simulink model "fuelcell"  (R2022b)
settings: Solver=VariableStepAuto  StartTime=0.0  StopTime=10720  RelTol=1e-2
model workspace (MAT data in the model file):
  N_P0 = 3
libraries: nesl_utility x7, sdl_lib x6, autolibshared x2, fl_lib x2, autolibrcnetworksystem x1, autolibmappedmotor x1
settings Model: Creator=connl  LastModifiedBy=user
settings SolverCC: MaxConsecutiveMinStep=5  DaesscMode=Robust  ZeroCrossAlgorithm=Adaptive  SolverResetMethod=Robust
settings DebuggingCC: AlgebraicLoopMsg=none  IgnoredZcDiagnostic=none

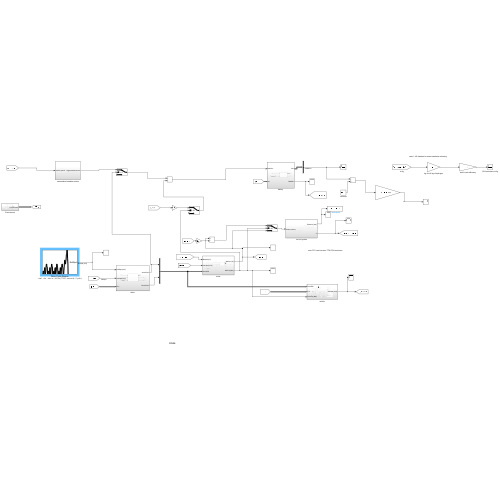
[thumbnail: Simulink's stored preview of the top-level diagram]
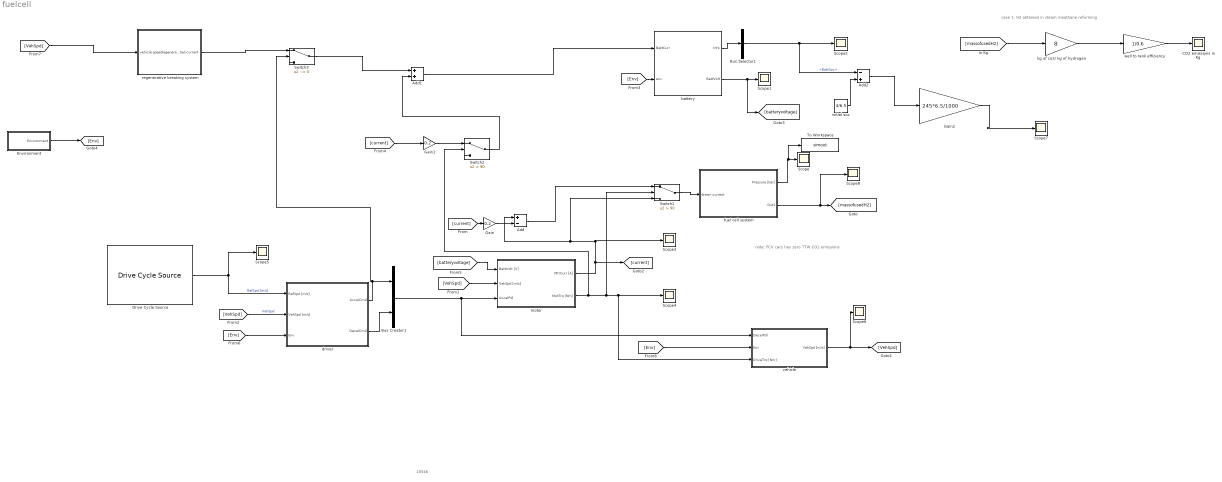
== system fuelcell ==
  note: 10546
  note: case 1: H2 obtained in steam meathane reforming
  note: note: FCV cars has zero TTW CO2 emissions
  Add : Sum  Inputs=+-
  Add1 : Sum
  Add2 : Sum  Inputs=-+
  Bus Creator1 : BusCreator  Inputs=2
  Bus Selector1 : BusSelector  OutputSignals=BattSoc
  CO2 emissions in Kg : Scope
  Drive Cycle Source : autolibshared/Drive Cycle Source  cycleVar=.mat, .xls, .xlsx or .txt file  wsVar=NEDC  fileVar=C:\Users\user\Desktop\my files\weekly meeting\drive cycles\NEDC.mat  tfinal="1180  seconds, Cyclic"  cycleRepeat=on  outAccPort=off  outGearPort=off  gearList=No gear data  t_wot1=5  xdot_woto=0  xdot_wot1=30  t_wot2=20  xdot_wot2=0  t_wotend=30  srcUnit=km/hr  outUnit=m/s  srcAccUnit=m/s/s  outAccUnit=m/s^2  dt=0  aMode=1  faultOption=off  velBnd=2  velBndUnit=mph  inUnit=m/s  timeBnd=1  failOption=off  stopSim=off  maxFaultCnt=10  maxFaultTime=2  maxTotFaultTime=15  traceOption=off  dtTrace=1  traceWindow=10  lastDCname=Custom Data Set 1  lastOutUnit=mph  lastDT=0  lastTB=1  lastSB=2  forceCalcBound=off
  Environment : Subsystem
  Gain : Gain  Gain=0.2
  Gain1 : Gain  Gain=0.2
  Gain2 : Gain  Gain=245*6.5/1000
  Scope{,1..8} (9 alike) : Scope
  Switch1 : Switch  Criteria=u2 > Threshold  Threshold=90  SaturateOnIntegerOverflow=off  InputSameDT=off
  Switch2 : Switch  Criteria=u2 > Threshold  Threshold=90  SaturateOnIntegerOverflow=off  InputSameDT=off
  Switch3 : Switch  Criteria=u2 ~= 0  SaturateOnIntegerOverflow=off  InputSameDT=off
  To Workspace : ToWorkspace  VariableName=simout  SaveFormat=Structure With Time  SampleTime=-1
  battery : Subsystem
  driver : Subsystem
  fuel cell system : Subsystem
  initial soc : Constant  Value=4/6.5
  kg of co2/ kg of hydrogen : Gain  Gain=8
  motor : Subsystem
  regenerative breaking system : Subsystem
  vehicle : Subsystem
  well to tank efficiency : Gain  Gain=1/0.6
  wires:
  Drive Cycle Source/1 -> Scope5/1, driver/1(RefSpd [m/s])  "RefSpd [m/s]"
  [VehSpd] -> driver/2(VehSpd [m/s])  "VehSpd"
  Bus Creator1/1 -> motor/3(AccelPdl), vehicle/1(DecelPdl)
  Environment/1(Environment) -> [Env]
  driver/2(DecelCmd) -> Bus Creator1/2
  driver/1(AccelCmd) -> Bus Creator1/1, Switch3/2
  [Env] -> driver/3(Env)
  fuel cell system/1(Pressure [bar]) -> To Workspace/1, Scope/1
  vehicle/1(VehSpd [m/s]) -> Scope6/1, [VehSpd]
  [Env] -> vehicle/2(Env)
  motor/2(MotTrq [Nm]) -> Switch1/2, Scope4/1, vehicle/3(DriveTrq [Nm]), Switch2/2
  [batteryvoltage] -> motor/1(BattVolt [V])
  [VehSpd] -> motor/2(VehSpd [m/s])
  [Env] -> battery/2(env)
  battery/1(Info) -> Bus Selector1/1
  motor/1(MtrCurr [A]) -> [current], Switch1/3, Add/1, Scope3/1
  Switch1/1 -> fuel cell system/1(drawn current)
  Add/1 -> Switch1/1
  Gain/1 -> Add/2
  Bus Selector1/1 -> Add2/1, Scope2/1  "<BattSoc>"
  [current] -> Gain/1
  [current] -> Gain1/1
  Gain1/1 -> Switch2/1
  Switch2/1 -> Add1/2
  [VehSpd] -> regenerative breaking system/1(vehicle speed)
  Switch3/1 -> Add1/1
  battery/2(BattVolt) -> [batteryvoltage], Scope1/1
  kg of co2/ kg of hydrogen/1 -> well to tank efficiency/1
  fuel cell system/2(Out1) -> Scope8/1, [massofusedH2]
  Add1/1 -> battery/1(BattCurr)
  well to tank efficiency/1 -> CO2 emissions in Kg/1
  [massofusedH2] -> kg of co2/ kg of hydrogen/1
  Add2/1 -> Gain2/1
  initial soc/1 -> Add2/2
  Gain2/1 -> Scope7/1
  regenerative breaking system/1(regenerated current) -> Switch3/1

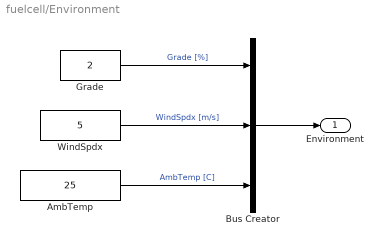
== system fuelcell/Environment ==
  AmbTemp : Constant  Value=25
  Bus Creator : BusCreator  Inputs=3
  Grade : Constant  Value=2
  WindSpdx : Constant  Value=5
  Environment : Outport
  wires:
  Grade/1 -> Bus Creator/1  "Grade [%]"
  WindSpdx/1 -> Bus Creator/2  "WindSpdx [m/s]"
  AmbTemp/1 -> Bus Creator/3  "AmbTemp [C]"
  Bus Creator/1 -> Environment/1

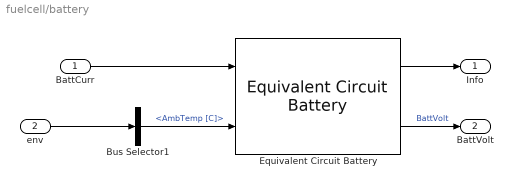
== system fuelcell/battery ==
  BattCurr : Inport
  env : Inport  Port=2
  Bus Selector1 : BusSelector  OutputSignals=AmbTemp [C]
  Equivalent Circuit Battery : autolibrcnetworksystem/Equivalent Circuit Battery  CapacityCtrl=Parameter  OutputVlt=Filtered  NumRC=1  Em=[245 245; 245 245]  R0=[0.011 0.11; 0.011 0.011]  SOC_BP=[0.5 1]  Temperature_BP=[293.15 313.15]  BattCap=[6.5 6.5]  BattCapInit=4  InitialCapVoltage=0  Tc=1/1000  Vinit=4.193  R1=[0.011 0.011; 0.011 0.011]  C1=|  R2=[0.011 0.011; 0.011 0.011]  C2=|  R3=[0.011 0.011; 0.011 0.011]  C3=|  R4=|  C4=|  R5=|  C5=|  Vu=Inf  Vl=-Inf  RefBlkName='autolibrcnetworksystem/Equivalent Circuit Battery'
      C1=|
      | [2287.7 11897;
      | 6122 24515]
      C2=|
      | [2287.7 11897;
      | 6122 24515]
      C3=|
      | [2287.7 11897;
      | 6122 24515]
      R4=|
      | [0.010342 0.0012244;
      | 0.0067316 0.0011396;
      | 0.0051156 0.0012661;
      | 0.0043447 0.0012265;
      | 0.0038826 0.0011163;
      | 0.0034226 0.0009968;
      | 0.003346 0.0011458;
      | 0.0033222 0.001345;
      | 0.0033201 0.0013091;
      | 0.0032886 0.0010986;
      | 0.0028114 0.0010309]
      C4=|
      | [2287.7 11897;
      | 6122 24515;
      | 18460 42098;
      | 20975 44453;
      | 15254 33098;
      | 10440 24492;
      | 13903 32975;
      | 16694 40007;
      | 15784 35937;
      | 12165 26430;
      | 9118 24795]
      R5=|
      | [0.010342 0.0012244;
      | 0.0067316 0.0011396;
      | 0.0051156 0.0012661;
      | 0.0043447 0.0012265;
      | 0.0038826 0.0011163;
      | 0.0034226 0.0009968;
      | 0.003346 0.0011458;
      | 0.0033222 0.001345;
      | 0.0033201 0.0013091;
      | 0.0032886 0.0010986;
      | 0.0028114 0.0010309]
      C5=|
      | [2287.7 11897;
      | 6122 24515;
      | 18460 42098;
      | 20975 44453;
      | 15254 33098;
      | 10440 24492;
      | 13903 32975;
      | 16694 40007;
      | 15784 35937;
      | 12165 26430;
      | 9118 24795]
  Info : Outport
  BattVolt : Outport  Port=2
  wires:
  Equivalent Circuit Battery/2 -> BattVolt/1  "BattVolt"
  env/1 -> Bus Selector1/1
  BattCurr/1 -> Equivalent Circuit Battery/1
  Equivalent Circuit Battery/1 -> Info/1
  Bus Selector1/1 -> Equivalent Circuit Battery/2  "<AmbTemp [C]>"

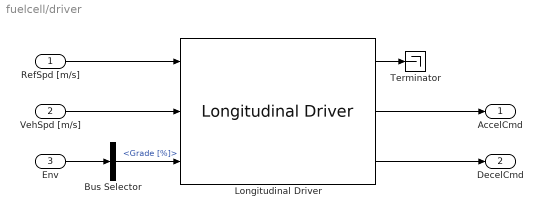
== system fuelcell/driver ==
  RefSpd [m/s] : Inport
  VehSpd [m/s] : Inport  Port=2
  Env : Inport  Port=3
  Bus Selector : BusSelector  OutputSignals=Grade [%]
  Longitudinal Driver : autolibshared/Longitudinal Driver  extAccelOvr=off  extDecelOvr=off  extAccelHld=off  extDecelHld=off  extAccelZero=off  extDecelZero=off  cntrlType=PI  shftType=None  velUnits=m/s  gearOut=off  Kp=10  Ki=2  Kff=0.05  Kg=0.01  VehVelVec=[0 100]  KffVec=[.1 .1]  KpVec=[10 10]  KiVec=[5 5]  KgVec=[0 0]  m=1500  Kpt=3000  tau=.1  L=2  aR=200  bR=2.5  cR=.5  g=9.81  vnom=100  Kaw=0.1  tauerr=0.03  tauPt=2  GearInit=0  tShift=.1  pdlVec=[0.1 0.4 0.5 0.9]  upShftTbl=[-1 12.9375 26.4375 39.9375 51.18749999999999 62.4375 72.84375 83.25;-1 16.3125 29.8125 43.3125 54.5624 65.8125 76.78125 87.75;-1 19.6875 33.1875 46.68749999999999 57.9375 69.1875 80.71875 92.25;-1 33 52.5 77.25 100.5 138.75 161.875 185]  dwnShftTbl=[1 9.5625 23.0625 36.5625 47.8125 59.0625 68.90625 78.75;1 12.9375 26.4375 39.9375 51.18749999999999 62.4375 72.84375 83.25;1 16.3125 29.8125 43.3125 54.562499 65.8125 76.78125 87.75;1 19.6875 33.1875 46.68749999999999 57.9375 69.1875 80.71875 92.25]  tClutch=.5  tRev=.5  tPark=120  aMode=1  UpGearVec="[0  1  2  3  4  5  6  7]"  DownGearVec="[1  2  3  4  5  6  7  8]"
  Terminator : Terminator
  AccelCmd : Outport
  DecelCmd : Outport  Port=2
  wires:
  Longitudinal Driver/1 -> Terminator/1
  Env/1 -> Bus Selector/1
  Bus Selector/1 -> Longitudinal Driver/3  "<Grade [%]>"
  RefSpd [m/s]/1 -> Longitudinal Driver/1
  VehSpd [m/s]/1 -> Longitudinal Driver/2
  Longitudinal Driver/3 -> DecelCmd/1
  Longitudinal Driver/2 -> AccelCmd/1

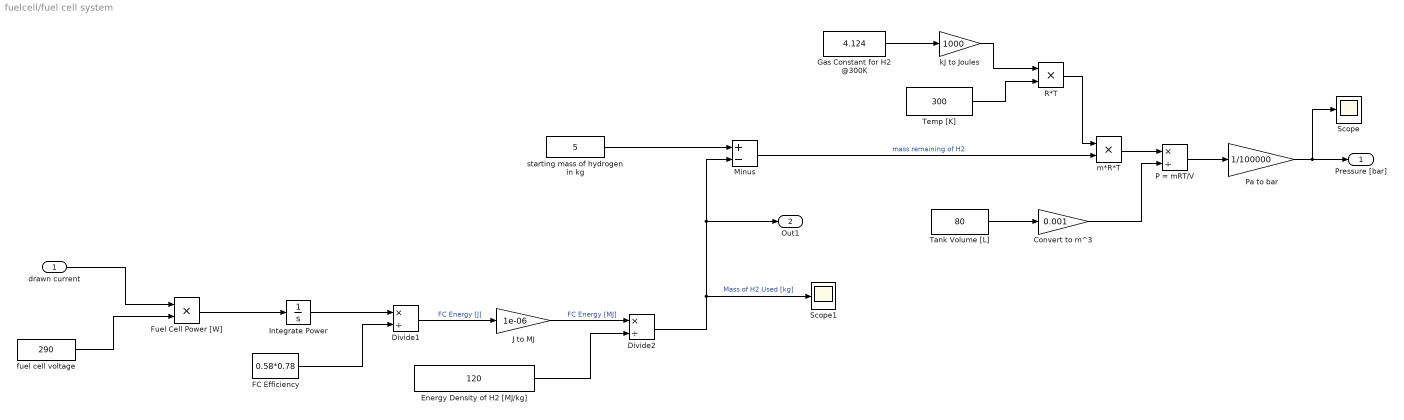
== system fuelcell/fuel cell system ==
  drawn current : Inport
  Convert to m^3 : Gain  Gain=0.001
  Divide1 : Product  Inputs=*/
  Divide2 : Product  Inputs=*/
  Energy Density of H2 [MJ/kg] : Constant  Value=120
  FC Efficiency : Constant  Value=0.58*0.78
  Fuel Cell Power [W] : Product
  Gas Constant for H2 @300K : Constant  Value=4.124
  Integrate Power : Integrator
  J to MJ : Gain  Gain=1e-06
  Minus : Sum  Inputs=+-
  P = mRT/V : Product  Inputs=*/
  Pa to bar : Gain  Gain=1/100000
  R*T : Product
  Scope : Scope
  Scope1 : Scope
  Tank Volume [L] : Constant  Value=80
  Temp [K] : Constant  Value=300
  fuel cell voltage : Constant  Value=290
  kJ to Joules : Gain  Gain=1000
  m*R*T : Product
  starting mass of hydrogen in kg : Constant  Value=5
  Pressure [bar] : Outport
  Out1 : Outport  Port=2
  wires:
  FC Efficiency/1 -> Divide1/2
  Integrate Power/1 -> Divide1/1
  m*R*T/1 -> P = mRT/V/1
  Pa to bar/1 -> Pressure [bar]/1, Scope/1
  P = mRT/V/1 -> Pa to bar/1
  fuel cell voltage/1 -> Fuel Cell Power [W]/2
  J to MJ/1 -> Divide2/1  "FC Energy [MJ]"
  drawn current/1 -> Fuel Cell Power [W]/1
  Gas Constant for H2 @300K/1 -> kJ to Joules/1
  Divide1/1 -> J to MJ/1  "FC Energy [J]"
  Minus/1 -> m*R*T/2  "mass remaining of H2"
  Divide2/1 -> Out1/1, Minus/2, Scope1/1  "Mass of H2 Used [kg]"
  kJ to Joules/1 -> R*T/1
  Convert to m^3/1 -> P = mRT/V/2
  R*T/1 -> m*R*T/1
  Tank Volume [L]/1 -> Convert to m^3/1
  Temp [K]/1 -> R*T/2
  Fuel Cell Power [W]/1 -> Integrate Power/1
  starting mass of hydrogen in kg/1 -> Minus/1
  Energy Density of H2 [MJ/kg]/1 -> Divide2/2

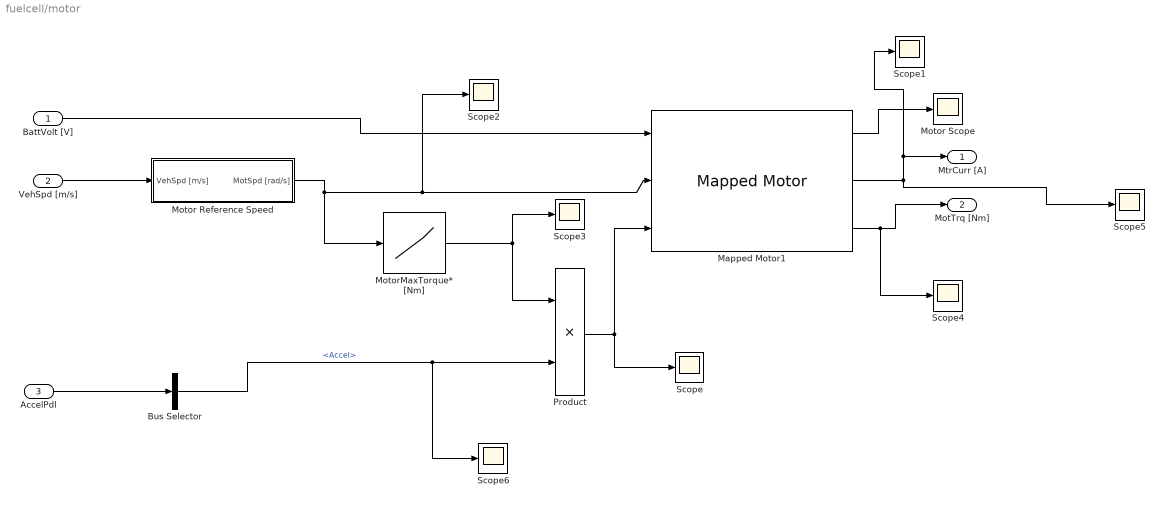
== system fuelcell/motor ==
  BattVolt [V] : Inport
  VehSpd [m/s] : Inport  Port=2
  AccelPdl : Inport  Port=3
  Bus Selector : BusSelector  OutputSignals=Accel
  Mapped Motor1 : autolibmappedmotor/Mapped Motor  port_config=Speed  param_by=Tabulated torque-speed envelope  w_t=[ 500 1000 1750 2000 3450]  T_t=[ 2494 1247 712 623 361]  torque_max=110  power_max=21000  Tc=0.02  param_loss=Single efficiency measurement  eff=90  w_eff=400  T_eff=55  Piron=0  Pbase=0  w_eff_bp=[-800 -400 0 400 800]  T_eff_bp=[0 0.03 0.06 0.09]  Temp_eff_bp=[233.15 293.15 373.15]  losses_table=[1.49 1.67 2.21 3.10; 0.42 0.69 1.14 2.03; 0.06 0.24 0.78 1.68; 0.42 0.69 1.14 2.03; 1.49 1.67 2.21 3.10]  losses_table_3d=cat(3,[1.49 1.67 2.21 3.10; 0.42 0.69 1.14 2.03; 0.06 0.24 0.78 1.68; 0.42 0.69 1.14 2.03; 1.49 1.67 2.21 3.10],[1.49 1.67 2.21 3.10; 0.42 0.69 1.14 2.03; 0.06 0.24 0.78 1.68; 0.42 0.69 1.14 2.03; 1.49 1.67 2.21 3.10],[1.49 1.67 2.21 3.10; 0.42 0.69 1.14 2.03; 0.06 0.24 0.78 1.68; 0.42 0.69 1.14 2.03; 1.49 1.67 2.21 3.10])  efficiency_table=[95 95 95 95; 95 95 95 95; 95 95 95 95; 95 95 95 95; 95 95 95 95]  efficiency_table_3d=cat(3,[95 95 95 95; 95 95 95 95; 95 95 95 95; 95 95 95 95; 95 95 95 95],[95 95 95 95; 95 95 95 95; 95 95 95 95; 95 95 95 95; 95 95 95 95],[95 95 95 95; 95 95 95 95; 95 95 95 95; 95 95 95 95; 95 95 95 95])  J=5e-6  b=1e-5  omega_o=0  T_t_extended=[361 623 712 1247 2494 2494 1247 712 623 361]  w_t_extended=[-3450 -2000 -1750 -1000 -500 500 1000 1750 2000 3450]  KLossIron=0  KLossCopper=0.80808  x_w_eff_vec=[-8000 -4000 0 4000 8000]  x_T_eff_vec=[-0.09 -0.06 -0.03 0 0.03 0.06 0.09]  x_tmp_eff_vec=[-0.09 -0.06 -0.03 0 0.03 0.06 0.09]  x_losses_mat=[3.1 2.21 1.67 1.49 1.67 2.21 3.1;2.03 1.14 0.69 0.42 0.69 1.14 2.03;1.68 0.78 0.24 0.06 0.24 0.78 1.68;2.03 1.14 0.69 0.42 0.69 1.14 2.03;3.1 2.21 1.67 1.49 1.67 2.21 3.1]  x_losses_mat_3d=[37.8947368421052 25.2631578947368 12.6315789473684 0 12 24 36;18.9473684210526 12.6315789473684 6.3157894736842 0 5.99999999999999 12 18;0 0 0 0 0 0 0;18 12 5.99999999999999 0 6.3157894736842 12.6315789473684 18.9473684210526;36 24 12 0 12.6315789473684 25.2631578947368 37.8947368421052]  CalLossMapData={}  CalLossWithTempMapData={}  aMode=1  RefBlkName='autolibmappedmotor/Mapped Motor'
  Motor Reference Speed : Subsystem
  Motor Scope : Scope
  MotorMaxTorque* [Nm] : Lookup_n-D  NumberOfTableDimensions=1  BreakpointsForDimension1=[ 500 1000 1750 2000 3450]  Table="[  2494 1247 712 623 361]"  InternalRulePriority=Speed  RndMeth=Simplest
  Product : Product
  Scope{,1..6} (7 alike) : Scope
  MtrCurr [A] : Outport
  MotTrq [Nm] : Outport  Port=2
  wires:
  Mapped Motor1/2 -> Scope1/1, MtrCurr [A]/1, Scope5/1
  Mapped Motor1/1 -> Motor Scope/1
  BattVolt [V]/1 -> Mapped Motor1/1
  Mapped Motor1/3 -> Scope4/1, MotTrq [Nm]/1
  Motor Reference Speed/1(MotSpd [rad/s]) -> Scope2/1, Mapped Motor1/2, MotorMaxTorque* [Nm]/1
  MotorMaxTorque* [Nm]/1 -> Product/1, Scope3/1
  VehSpd [m/s]/1 -> Motor Reference Speed/1(VehSpd [m/s])
  Bus Selector/1 -> Scope6/1, Product/2  "<Accel>"
  AccelPdl/1 -> Bus Selector/1
  Product/1 -> Mapped Motor1/3, Scope/1

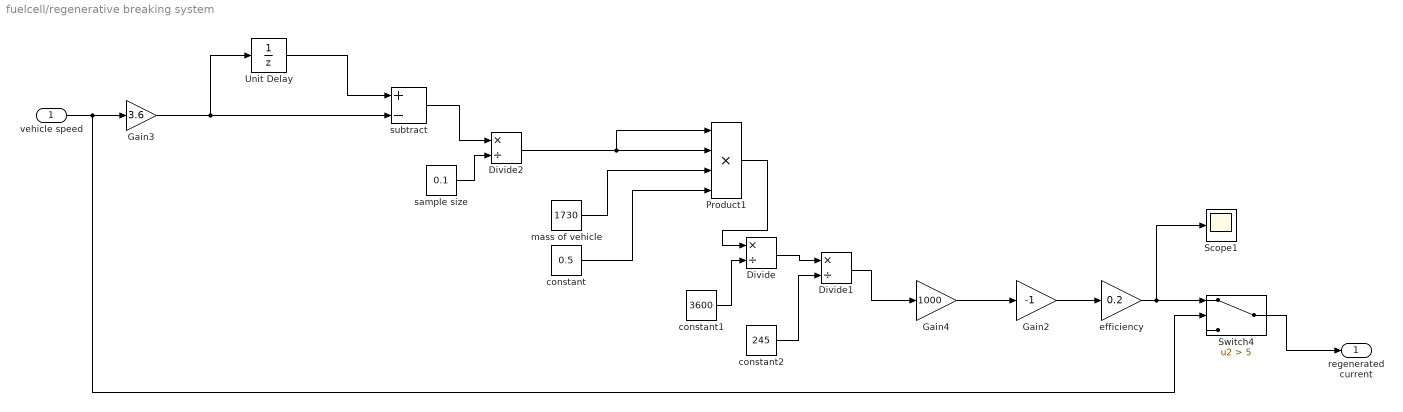
== system fuelcell/regenerative breaking system ==
  vehicle speed : Inport
  Divide : Product  Inputs=*/
  Divide1 : Product  Inputs=*/
  Divide2 : Product  Inputs=*/
  Gain2 : Gain  Gain=-1
  Gain3 : Gain  Gain=3.6
  Gain4 : Gain  Gain=1000
  Product1 : Product  Inputs=4
  Scope1 : Scope
  Switch4 : Switch  Criteria=u2 > Threshold  Threshold=5  SaturateOnIntegerOverflow=off  InputSameDT=off
  Unit Delay : UnitDelay  SampleTime=0.1  HasFrameUpgradeWarning=on
  constant : Constant  Value=0.5
  constant1 : Constant  Value=3600
  constant2 : Constant  Value=245
  efficiency : Gain  Gain=0.2
  mass of vehicle : Constant  Value=1730
  sample size : Constant  Value=0.1
  subtract : Sum  Inputs=+-
  regenerated current : Outport
  wires:
  constant1/1 -> Divide/2
  Divide1/1 -> Gain4/1
  constant2/1 -> Divide1/2
  mass of vehicle/1 -> Product1/3
  Gain3/1 -> subtract/2, Unit Delay/1
  Divide/1 -> Divide1/1
  Unit Delay/1 -> subtract/1
  constant/1 -> Product1/4
  Gain4/1 -> Gain2/1
  Switch4/1 -> regenerated current/1
  Gain2/1 -> efficiency/1
  efficiency/1 -> Scope1/1, Switch4/1
  Product1/1 -> Divide/1
  vehicle speed/1 -> Switch4/2, Gain3/1
  subtract/1 -> Divide2/1
  Divide2/1 -> Product1/2, Product1/1
  sample size/1 -> Divide2/2

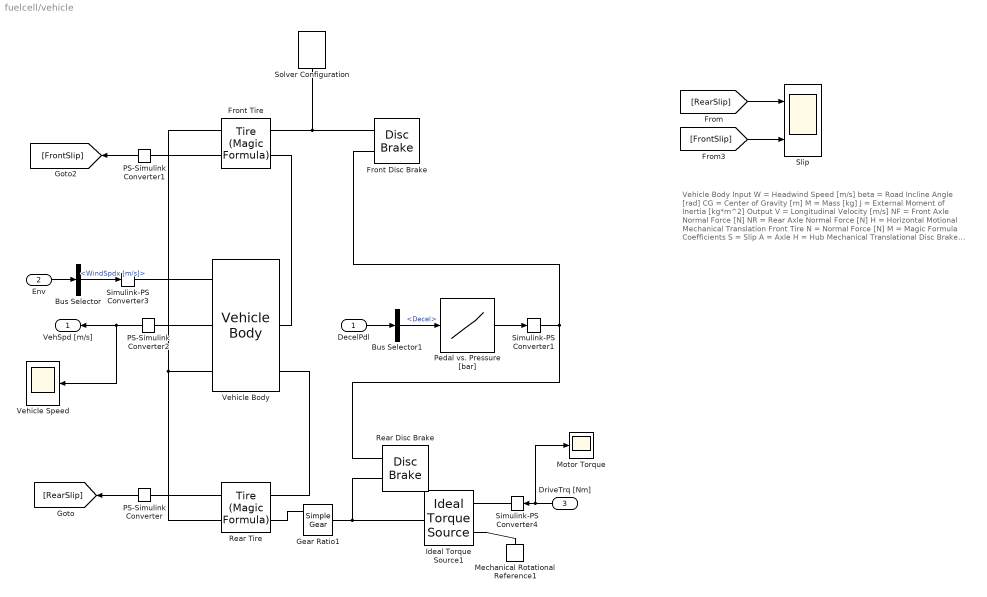
== system fuelcell/vehicle ==
  note: Vehicle Body
      | Input
      | W = Headwind Speed [m/s]
      | beta = Road Incline Angle [rad]
      | CG = Center of Gravity [m]
      | M = Mass [kg]
      | J = External Moment of Inertia [kg*m^2]
      |
      | Output
      | V = Longitudinal Velocity [m/s]
      | NF = Front Axle Normal Force [N]
      | NR = Rear Axle Normal Force [N]
      | H = Horizontal Motional Mechanical Translation
      |
      | Front Tire
      | N = Normal Force [N]
      | M = Magic Formula Coefficients
      | S = Slip
      | A = Axle
      | H = Hub Mechanical Translational
      |
      | Disc Brake
      | P = Cylinder Pressure [bars]
      | S = Shaft Rotational Mechanical
      |
      | Ideal Torque Source
      | S = Control Signal [Nm]
      | C = Case Mechanical Rotational with the Source Reference Point
      | R = Rod Mechanical Rotational Port with the Source Moving Part
  DecelPdl : Inport
  Env : Inport  Port=2
  DriveTrq [Nm] : Inport  Port=3
  Bus Selector : BusSelector  OutputSignals=WindSpdx [m/s]
  Bus Selector1 : BusSelector  OutputSignals=Decel
  Front Disc Brake : sdl_lib/Brakes & Detents/Rotational/Disc Brake  r_mean=0.05 m  bore=0.05 m  n_pads=2  thermal_port=simscape.enum.thermaleffects.omit  mu_static=0.1  mu_coulomb=0.1  temperature_TLU=[280, 300, 320] K  mu_static_TLU=[.9, .8, .7]  mu_coulomb_TLU=[.8, .7, .6]  brkwy_vel=0.1 rad/s  visc_coef=0.001 N*m/(rad/s)  enable_faults=simscape.enum.onoff.off  faulted_pressure=0 bar  external_fault=simscape.enum.onoff.off  temporal_fault=simscape.enum.onoff.off  fault_time=5 s  report_fault=simscape.enum.assert.action.none  thermal_mass=50 kJ/K  temperature_specify=off  temperature_priority=High  temperature=300 K  temperature_nominal_specify=off  temperature_nominal_unit=K  temperature_nominal_value=1
  Front Tire : sdl_lib/Tires & Vehicles/Tire (Magic Formula)  parameterization=sdl.enum.magic_tire_model.peak  F_z1=30000 N  F_x1=35000 N  kappa1=6  B_m=10  C_m=1.9  D_m=1  E_m=0.97  fz0=4e+3 N  p_Cx=1.685  p_Dx=[ 1.21 -0.037 ]  p_Ex=[ 0.344 0.095 -0.02 0 ]  p_Kx=[ 21.51 -0.163 0.245 ]  p_Hx=[ -0.002 0.002 ]  p_Vx=[ 0 0 ]  r_e=0.316 m  model_compliance=0  stiffness=1e+6 N/m  damping=1000 N/(m/s)  model_inertia=1  inertia=1.02 kg*m^2  initial_velocity=0 rad/s  model_resistance=1  resistance_model=1  coeff=0.03  p_tire=250e3 Pa  alpha=-0.003  beta=0.97  coeff_a=84e-4  coeff_b=6.2e-4 s/m  coeff_c=1.6e-4 s^2/m^2  v_thr=1e-3 m/s  v_tr_thr=0.1*(0.1) m/s
  Gear Ratio1 : sdl_lib/Gears/Simple Gear  ratio=1/6  rotation_direction=sdl.enum.shaftOutputDirection.same  friction_model=sdl.enum.gear_efficiencies_load.temperatureLoad  T_noload=0.1 N*m  T_nom=5 N*m  efficiency_nom=0.8  efficiency=0.8  temperature_TLU=[280, 300, 320] K  load_TLU=[1, 5, 10] N*m  efficiency_TLU=[.95, .9, .85]  efficiency_TLU2=[.85, .8, .75; .95, .9, .85; .85, .8, .7]  w_thr=0.01 rad/s  pwr_thr=0.001 W  backlash_model=sdl.enum.backlashModel.Off  backlash_distance=1e-3 mm  x0=0 mm  r_base=0.1 m  hardstop_model=simscape.enum.hardstop.smooth  transition=1e-4 mm  backlash_stiffness=1e6 N/m  backlash_damping=1e3 N*s/m  e=0  v_tol=0.001 m/s  mu_visc=[0, 0] N*m*s/rad  enable_faults=simscape.enum.onoff.off  efficiency_fault=0.05  external_fault=simscape.enum.onoff.off  temporal_fault=simscape.enum.onoff.off  fault_time=5 s  fault_angles=pi / 12 rad  report_fault=simscape.enum.assert.action.none  thermal_mass=50 J/K  temperature_specify=off  temperature_priority=High  temperature=300 K  temperature_nominal_specify=off  temperature_nominal_unit=K  temperature_nominal_value=1  x_backlash_specify=off  x_backlash_priority=None  x_backlash=0 mm  x_backlash_nominal_specify=off  x_backlash_nominal_unit=mm  x_backlash_nominal_value=1  f_hardstop_specify=off  f_hardstop_priority=None  f_hardstop=0 N  f_hardstop_nominal_specify=off  f_hardstop_nominal_unit=N  f_hardstop_nominal_value=1  v_backlash_specify=off  v_backlash_priority=None  v_backlash=0 m/s  v_backlash_nominal_specify=off  v_backlash_nominal_unit=m/s  v_backlash_nominal_value=1
      settings: InternalSimscapePortConfiguration="{\"Bottom\":[],\"Left\":[{\"id\":\"B\",\"label\":\"B\",\"type\":\"foundation.mechanical.rotational.rotational\"},{\"id\":\"H\",\"label\":\"H\",\"type\":\"foundation.thermal.thermal\"}],\"Right\":[{\"id\":\"F\",\"label\":\"F\",\"type\":\"foundation.mechanical.rotational.rotational\"}],\"Top\":[]}"
  Ideal Torque Source1 : fl_lib/Mechanical/Mechanical Sources/Ideal Torque Source
  Mechanical Rotational Reference1 : fl_lib/Mechanical/Rotational Elements/Mechanical Rotational Reference
  Motor Torque : Scope
  PS-Simulink Converter : nesl_utility/PS-Simulink Converter  PhysicalDomain=network_engine_domain  SubClassName=ps_output  LeftPortType=input  RightPortType=output  PseudoPeriodic=off  Frequencies=[]  VectorFormat=inherit  Unit=inherit  AffineConversion=off
  PS-Simulink Converter1 : nesl_utility/PS-Simulink Converter  PhysicalDomain=network_engine_domain  SubClassName=ps_output  LeftPortType=input  RightPortType=output  PseudoPeriodic=off  Frequencies=[]  VectorFormat=inherit  Unit=inherit  AffineConversion=off
  PS-Simulink Converter2 : nesl_utility/PS-Simulink Converter  PhysicalDomain=network_engine_domain  SubClassName=ps_output  LeftPortType=input  RightPortType=output  PseudoPeriodic=off  Frequencies=[]  VectorFormat=inherit  Unit=m/s  AffineConversion=off
  Pedal vs. Pressure [bar] : Lookup_n-D  NumberOfTableDimensions=1  BreakpointsForDimension1=[-5:5]  Table=tanh([-5:5])  InternalRulePriority=Speed  RndMeth=Simplest
  Rear Disc Brake : sdl_lib/Brakes & Detents/Rotational/Disc Brake  r_mean=0.05 m  bore=0.05 m  n_pads=2  thermal_port=simscape.enum.thermaleffects.omit  mu_static=0.1  mu_coulomb=0.1  temperature_TLU=[280, 300, 320] K  mu_static_TLU=[.9, .8, .7]  mu_coulomb_TLU=[.8, .7, .6]  brkwy_vel=0.1 rad/s  visc_coef=0.001 N*m/(rad/s)  enable_faults=simscape.enum.onoff.off  faulted_pressure=0 bar  external_fault=simscape.enum.onoff.off  temporal_fault=simscape.enum.onoff.off  fault_time=5 s  report_fault=simscape.enum.assert.action.none  thermal_mass=50 kJ/K  temperature_specify=off  temperature_priority=High  temperature=300 K  temperature_nominal_specify=off  temperature_nominal_unit=K  temperature_nominal_value=1
  Rear Tire : sdl_lib/Tires & Vehicles/Tire (Magic Formula)  parameterization=1  F_z1=30000 N  F_x1=30000 N  kappa1=6  B_m=10  C_m=1.9  D_m=1  E_m=0.97  fz0=4e+3 N  p_Cx=1.685  p_Dx=[ 1.21 -0.037 ]  p_Ex=[ 0.344 0.095 -0.02 0 ]  p_Kx=[ 21.51 -0.163 0.245 ]  p_Hx=[ -0.002 0.002 ]  p_Vx=[ 0 0 ]  r_e=0.316 m  model_compliance=0  stiffness=1e+6 N/m  damping=1000 N/(m/s)  model_inertia=1  inertia=1.02 kg*m^2  initial_velocity=0 rad/s  model_resistance=1  resistance_model=1  coeff=0.03  p_tire=250e3 Pa  alpha=-0.003  beta=0.97  coeff_a=84e-4  coeff_b=6.2e-4 s/m  coeff_c=1.6e-4 s^2/m^2  v_thr=1e-3 m/s  v_tr_thr=0.1*(0.1) m/s
  Simulink-PS Converter1 : nesl_utility/Simulink-PS Converter  PhysicalDomain=network_engine_domain  SubClassName=ps_input  LeftPortType=input  RightPortType=output  PseudoPeriodic=off  Frequencies=[]  NoiseDistribution=none  NoiseParameters=[]  Unit=bar  AffineConversion=off  FilteringAndDerivatives=provide  SimscapeFilterOrder=1  InputFilterTimeConstant=0.01  UdotUserProvided=0
  Simulink-PS Converter3 : nesl_utility/Simulink-PS Converter  PhysicalDomain=network_engine_domain  SubClassName=ps_input  LeftPortType=input  RightPortType=output  PseudoPeriodic=off  Frequencies=[]  NoiseDistribution=none  NoiseParameters=[]  Unit=m/s  AffineConversion=off  FilteringAndDerivatives=provide  SimscapeFilterOrder=1  InputFilterTimeConstant=0.01  UdotUserProvided=0
  Simulink-PS Converter4 : nesl_utility/Simulink-PS Converter  PhysicalDomain=network_engine_domain  SubClassName=ps_input  LeftPortType=input  RightPortType=output  PseudoPeriodic=off  Frequencies=[]  NoiseDistribution=none  NoiseParameters=[]  Unit=N*m  AffineConversion=off  FilteringAndDerivatives=provide  SimscapeFilterOrder=1  InputFilterTimeConstant=0.01  UdotUserProvided=0
  Slip : Scope  NumInputPorts=2
  Solver Configuration : nesl_utility/Solver Configuration  PhysicalDomain=network_engine_domain  SubClassName=solver  LeftPortType=input  RightPortType=generic  Tones=[]  Harmonics=[]  SimulateNoise=off  Profile=off  UseLocalSampling=off  EnableSwitchedLinearOptims=on  FrequencyDomain=off  UseCCode=off  RelTol=0.001  AbsTol=0.001  MinStep=1e-09  ToWorkspace=off  RevertToSquareIcSolve=off  NumHomotopyIterations=100  PhasorMode=off  PhasorModeNumHarmonics=1  ConsistencySolver=NEWTON_XTOL_AFTER_FTOL  IndexReductionMethod=DerivativeReplacement  DoDC=off  ResidualTolerance=1e-09  ConsistencyTolSource=GLOBAL  ConsistencyAbsTol=0.001  ConsistencyRelTol=0.001  ConsistencyTolFactor=0.001  UseLocalSolver=off  LocalSolverChoice=NE_BACKWARD_EULER_ADVANCER  ResolveIndetEquations=on  FunctionEvalNumThread=1  LocalSolverSampleTime=0.001  DoFixedCost=off  MaxNonlinIter=3  MaxModeIter=2  ComputeImpulses=off  ImpulseIterations=2  LinearAlgebra=auto  LinearAlgebraNumThread=0  EquationFormulation=NE_TIME_EF  DelaysMemoryBudget=1024  AutomaticFiltering=on  FilteringTimeConstant=0.001  PartitionStorageMethod=AS_NEEDED  PartitionMemoryBudget=1024  PartitionMethod=ROBUST
  Vehicle Body : sdl_lib/Tires & Vehicles/Vehicle Body  mass=1719 kg  n_w=1  x_f=1.195 m  x_r=1.513 m  y_c=0.5 m  mass_var=simscape.enum.onoff.off  g=9.81 m/s^2  liftoff_warning=0  area=2.31 m^2  Cd=0.314  rho=1.3 kg/m^3  model_pitch=simscape.enum.onoff.off  inertia=4000 kg*m^2  suspension_model=1  k_f=1e4 N/m  b_f=1e4 N/(m/s)  k_r=1e4 N/m  b_r=1e4 N/(m/s)  k_f_TLU=[-2000, -1000, 0, 1000, 2000] N  x_f_TLU=[-.4, -.2, 0, .2, .4] m  b_f_TLU=[-200, -100, 0, 100, 200] N  v_f_TLU=[-4, -2, 0, 2, 4] m/s  k_r_TLU=[-2000, -1000, 0, 1000, 2000] N  x_r_TLU=[-.4, -.2, 0, .2, .4] m  b_r_TLU=[-200, -100, 0, 100, 200] N  v_r_TLU=[-4, -2, 0, 2, 4] m/s  interp_method=simscape.enum.interpolation.linear  extrap_method=simscape.enum.extrapolation.linear  model_hardstop=0  upper_bound_f=.25 m  lower_bound_f=-.25 m  stop_k_f=1e6 N/m  stop_b_f=150 N/(m/s)  upper_bound_r=.25 m  lower_bound_r=-.25 m  stop_k_r=1e6 N/m  stop_b_r=150 N/(m/s)  initial_pitch=0 rad  initial_pitch_rate=0 rad/s  v_specify=on  v_priority=High  v=0 m/s  v_nominal_specify=off  v_nominal_unit=m/s  v_nominal_value=1
  Vehicle Speed : Scope
  VehSpd [m/s] : Outport
  wires:
  DriveTrq [Nm]/1 -> Motor Torque/1, Simulink-PS Converter4/1
  [FrontSlip] -> Slip/2
  Pedal vs. Pressure [bar]/1 -> Simulink-PS Converter1/1
  PS-Simulink Converter2/1 -> VehSpd [m/s]/1, Vehicle Speed/1
  [RearSlip] -> Slip/1
  Bus Selector1/1 -> Pedal vs. Pressure [bar]/1  "<Decel>"
  Bus Selector/1 -> Simulink-PS Converter3/1  "<WindSpdx [m/s]>"
  PS-Simulink Converter/1 -> [RearSlip]
  Env/1 -> Bus Selector/1
  PS-Simulink Converter1/1 -> [FrontSlip]
  DecelPdl/1 -> Bus Selector1/1
  connections:
  Simulink-PS Converter3/RConn1 -- Vehicle Body/LConn3
  Rear Tire/LConn2 -- Gear Ratio1/LConn1
  Vehicle Body/RConn1 -- Rear Tire/LConn1
  Ideal Torque Source1/RConn2 -- Mechanical Rotational Reference1/LConn1
  Front Tire/RConn1 -- PS-Simulink Converter1/LConn1
  Front Tire/RConn2 -- Vehicle Body/LConn1 -- Rear Tire/RConn2
  Ideal Torque Source1/RConn1 -- Simulink-PS Converter4/RConn1
  Front Disc Brake/LConn1 -- Simulink-PS Converter1/RConn1 -- Rear Disc Brake/LConn1
  Rear Disc Brake/LConn2 -- Gear Ratio1/RConn1 -- Ideal Torque Source1/LConn1
  Vehicle Body/LConn2 -- PS-Simulink Converter2/LConn1
  Front Tire/LConn2 -- Front Disc Brake/LConn2 -- Solver Configuration/RConn1
  Rear Tire/RConn1 -- PS-Simulink Converter/LConn1
  Vehicle Body/RConn2 -- Front Tire/LConn1

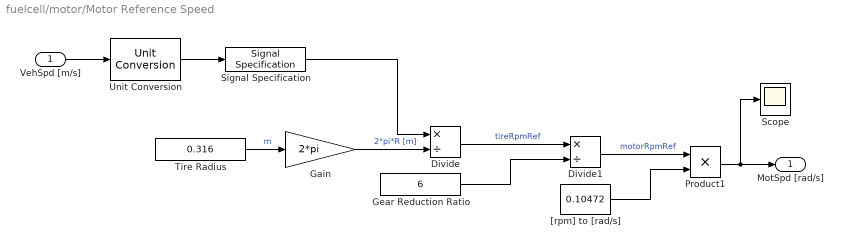
== system fuelcell/motor/Motor Reference Speed ==
  VehSpd [m/s] : Inport
  Divide : Product  Inputs=*/
  Divide1 : Product  Inputs=*/
  Gain : Gain  Gain=2*pi
  Gear Reduction Ratio : Constant  Value=6
  Product1 : Product
  Scope : Scope
  Signal Specification : SignalSpecification  Unit=m/min
  Tire Radius : Constant  Value=0.316
  Unit Conversion : UnitConversion
  "[rpm] to [rad/s]" : Constant  Value=0.10472
  MotSpd [rad/s] : Outport
  wires:
  VehSpd [m/s]/1 -> Unit Conversion/1
  Divide/1 -> Divide1/1  "tireRpmRef"
  Gain/1 -> Divide/2  "2*pi*R [m]"
  Gear Reduction Ratio/1 -> Divide1/2
  Tire Radius/1 -> Gain/1  "m"
  Product1/1 -> MotSpd [rad/s]/1, Scope/1
  "[rpm] to [rad/s]"/1 -> Product1/2
  Divide1/1 -> Product1/1  "motorRpmRef"
  Signal Specification/1 -> Divide/1
  Unit Conversion/1 -> Signal Specification/1
